simulink library "ss_angles_2_vec"  (R2016b)
settings: Solver=VariableStepAuto  StartTime=0.0  StopTime=10.0  RelTol=1e-3
settings Model: Creator=taylorreynolds  LastModifiedBy=Taylor

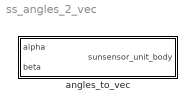
== system ss_angles_2_vec ==
  angles_to_vec : Subsystem

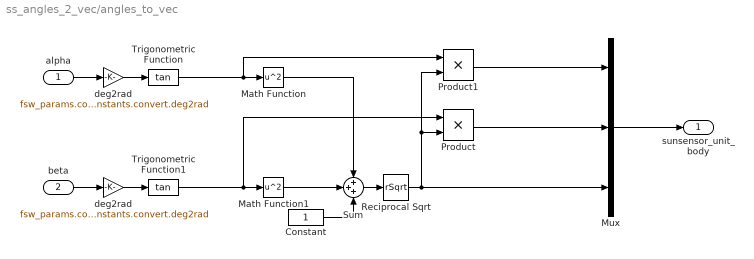
== system ss_angles_2_vec/angles_to_vec ==
  alpha : Inport
  beta : Inport  Port=2
  Constant : Constant
  Math Function : Math  Operator=square  SaturateOnIntegerOverflow=on
  Math Function1 : Math  Operator=square  SaturateOnIntegerOverflow=on
  Mux : Mux  Inputs=3
  Product : Product
  Product1 : Product
  Reciprocal Sqrt : Sqrt  Operator=rSqrt  SaturateOnIntegerOverflow=on
  Sum : Sum  Inputs=+++
  Trigonometric Function : Trigonometry  Operator=tan  OutputSignalType=real
  Trigonometric Function1 : Trigonometry  Operator=tan  OutputSignalType=real
  deg2rad : Gain  Gain=fsw_params.constants.convert.deg2rad
  "deg2rad " : Gain  Gain=fsw_params.constants.convert.deg2rad
  sunsensor_unit_body : Outport
  wires:
  beta/1 -> "deg2rad "/1
  alpha/1 -> deg2rad/1
  Product1/1 -> Mux/1
  Product/1 -> Mux/2
  Reciprocal Sqrt/1 -> Mux/3, Product/2, Product1/2
  Mux/1 -> sunsensor_unit_body/1
  deg2rad/1 -> Trigonometric Function/1
  "deg2rad "/1 -> Trigonometric Function1/1
  Trigonometric Function/1 -> Product1/1, Math Function/1
  Trigonometric Function1/1 -> Product/1, Math Function1/1
  Sum/1 -> Reciprocal Sqrt/1
  Constant/1 -> Sum/3
  Math Function1/1 -> Sum/2
  Math Function/1 -> Sum/1
